simulink model "FPA_sincos_subsystem_template"  (R2016a)
settings: Solver=ode45  StartTime=0.0  StopTime=10.0  RelTol=1e-3
libraries: simulink x3
settings Model: Creator=cliu  LastModifiedBy=bzhuang
settings DataIOCC: LimitDataPoints=on  SaveFormat=Array  SignalLoggingSaveFormat=ModelDataLogs
settings OptimizationCC: ExpressionDepthLimit=2147483647
settings DebuggingCC: UnderspecifiedInitializationDetection=Classic  MergeDetectMultiDrivingBlocksExec=none  SolverPrmCheckMsg=warning  FcnCallInpInsideContextMsg=UseLocalSettings  StateNameClashWarn=warning  StrictBusMsg=Warning
settings HardwareCC: ProdBitPerPointer=32  ProdLargestAtomicFloat=None  ProdIntDivRoundTo=Undefined  ProdEndianess=Unspecified  ProdWordSize=32  ProdHWDeviceType=32-bit Generic
settings ModelReferenceCC: PropagateSignalLabelsOutOfModel=off
settings GRTTargetCC: UseEC=on  UseSLC=on  CombineOutputUpdateFcns=off  GRTInterface=on
settings ConfigComp: CovModelRefEnable=Off

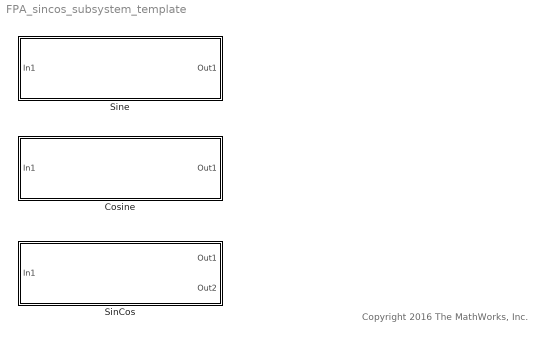
== system FPA_sincos_subsystem_template ==
  note: Copyright 2016 The MathWorks, Inc.
  Cosine : Subsystem
  SinCos : Subsystem
  Sine : Subsystem

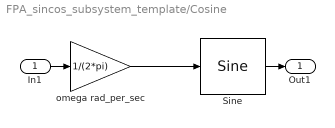
== system FPA_sincos_subsystem_template/Cosine ==
  In1 : Inport
  Sine : simulink/Lookup Tables/Sine  Formula=cos(2*pi*u)  NumDataPoints=(2^5)+1  OutputWordLength=16  InternalRulePriority=Speed
  omega rad_per_sec : Gain  Gain=1/(2*pi)  ParamDataTypeStr=Inherit: Same as input
  Out1 : Outport
  wires:
  omega rad_per_sec/1 -> Sine/1
  Sine/1 -> Out1/1
  In1/1 -> omega rad_per_sec/1

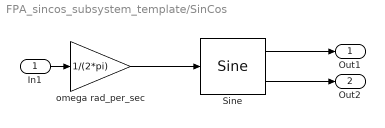
== system FPA_sincos_subsystem_template/SinCos ==
  In1 : Inport
  Sine : simulink/Lookup Tables/Sine  Formula=sin(2*pi*u) and cos(2*pi*u)  NumDataPoints=(2^5)+1  OutputWordLength=16  InternalRulePriority=Speed
  omega rad_per_sec : Gain  Gain=1/(2*pi)  ParamDataTypeStr=Inherit: Same as input
  Out1 : Outport
  Out2 : Outport  Port=2
  wires:
  omega rad_per_sec/1 -> Sine/1
  Sine/1 -> Out1/1
  In1/1 -> omega rad_per_sec/1
  Sine/2 -> Out2/1

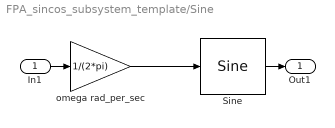
== system FPA_sincos_subsystem_template/Sine ==
  In1 : Inport
  Sine : simulink/Lookup Tables/Sine  Formula=sin(2*pi*u)  NumDataPoints=(2^5)+1  OutputWordLength=16  InternalRulePriority=Speed
  omega rad_per_sec : Gain  Gain=1/(2*pi)  ParamDataTypeStr=Inherit: Same as input
  Out1 : Outport
  wires:
  omega rad_per_sec/1 -> Sine/1
  Sine/1 -> Out1/1
  In1/1 -> omega rad_per_sec/1
